simulink model "karimi5"  (Simulink 7.1)
settings: Solver=ode45  StartTime=0.0  StopTime=10.0  RelTol=1e-3
libraries: powerlib_extras x2
settings Model: Creator=m  LastModifiedBy=m

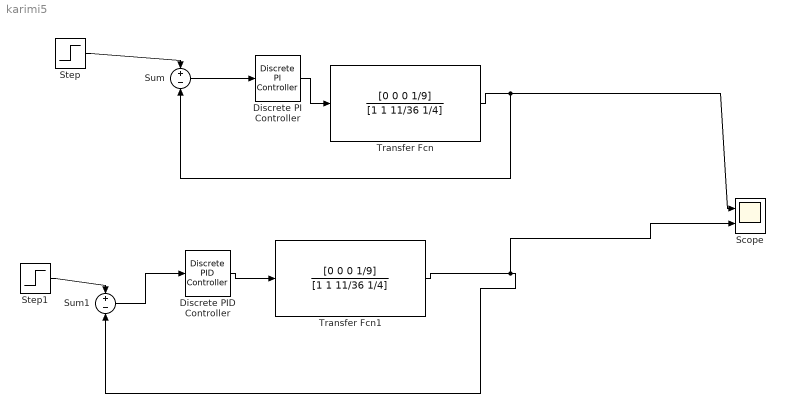
== system karimi5 ==
  Discrete PI Controller : powerlib_extras/Discrete  Control Blocks/Discrete PI Controller  DialogController=POWERSYS.PowerSysDialog  SystemSampleTime=-1  Kp=1.14  Ki=9.475  Par_Limits=[1e6 -1e6]  Init=0  Ts=50e-6
  Discrete PID Controller : powerlib_extras/Discrete  Control Blocks/Discrete PID Controller  DialogController=POWERSYS.PowerSysDialog  SystemSampleTime=-1  Kp=1.47  Ki=5.865  Kd=1.421  TcD=1  Par_Limits=[100 -100]  Init=0  Ts=0.5
  Scope : Scope  NumInputPorts=2
      settings: TimeRange=10  YMin=-32.6~-14  YMax=-30.6~-10.5
  Step : Step  SampleTime=0  VectorParams1D=off  ZeroCross=off
  Step1 : Step  SampleTime=0  VectorParams1D=off  ZeroCross=off
  Sum : Sum  Inputs=+-  OutDataType=sfix(16)  OutScaling=2^0
  Sum1 : Sum  Inputs=+-  OutDataType=sfix(16)  OutScaling=2^0
  Transfer Fcn : TransferFcn  Numerator=[0 0 0 1/9]  Denominator=[1 1 11/36 1/4]
  Transfer Fcn1 : TransferFcn  Numerator=[0 0 0 1/9]  Denominator=[1 1 11/36 1/4]
  wires:
  Step/1 -> Sum/1
  Sum/1 -> Discrete PI Controller/1
  Discrete PI Controller/1 -> Transfer Fcn/1
  Transfer Fcn/1 -> Sum/2, Scope/1
  Discrete PID Controller/1 -> Transfer Fcn1/1
  Step1/1 -> Sum1/1
  Sum1/1 -> Discrete PID Controller/1
  Transfer Fcn1/1 -> Sum1/2, Scope/2
